simulink model "sin_w_st"  (R2022b)
settings: Solver=ode5  StartTime=0.0  StopTime=t_s  FixedStep=h  RelTol=1e-3
undefined symbols (not defined in the file): A, f
settings Model: Creator=Claudia Yasar  LastModifiedBy=Claudia Yasar
settings DataIOCC: ReturnWorkspaceOutputs=off

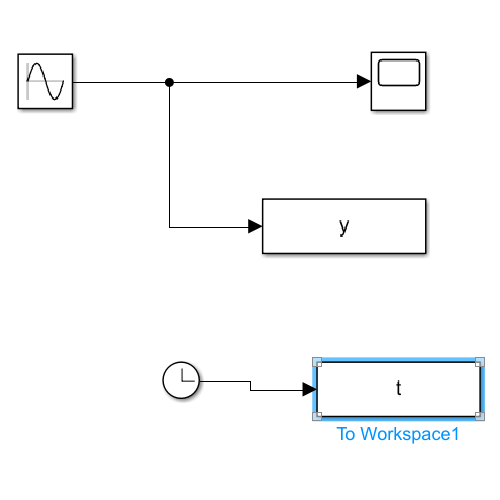
[thumbnail: Simulink's stored preview of the top-level diagram]
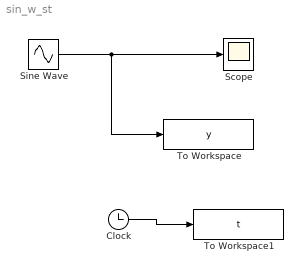
== system sin_w_st ==
  Clock : Clock
  Scope : Scope
  Sine Wave : Sin  Amplitude=A  Frequency=f  SampleTime=0
  To Workspace : ToWorkspace  VariableName=y  SampleTime=-1
  To Workspace1 : ToWorkspace  VariableName=t  SampleTime=-1
  wires:
  Sine Wave/1 -> To Workspace/1, Scope/1
  Clock/1 -> To Workspace1/1
